simulink model "Spring_OscillationExt"  (R2017b)
settings: Solver=FixedStepAuto  StartTime=0.0  StopTime=50.0  FixedStep=0.01  RelTol=1e-3
values from neighbouring files (symbols this model uses):
  k = k+26    [Caesarcipher.m]
  m = mean(r)    [plotrand.m]
undefined symbols (not defined in the file or in its folder): c
settings Model: Creator=Mahe  LastModifiedBy=Mahe

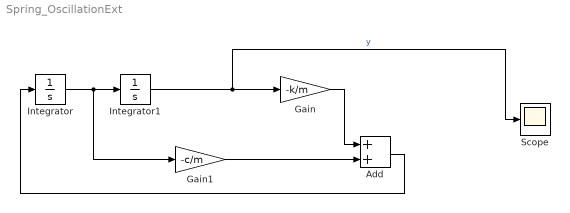
== system Spring_OscillationExt ==
  Add : Sum
  Gain : Gain  Gain=-k/m
  Gain1 : Gain  Gain=-c/m
  Integrator : Integrator
  Integrator1 : Integrator  InitialCondition=10
  Scope : Scope
  wires:
  Integrator/1 -> Gain1/1, Integrator1/1
  Integrator1/1 -> Scope/1, Gain/1  "y"
  Gain/1 -> Add/1
  Add/1 -> Integrator/1
  Gain1/1 -> Add/2
